simulink model "controller_test"  (R2015a)
settings: Solver=ode5  StartTime=0.0  StopTime=9  FixedStep=1e-4  RelTol=1e-3
values from neighbouring files (symbols this model uses):
  A = A(1:4,1:4)    [main_matlab_version_3.m]    (also in main_matlab_version_4.m)
  B = B(1:4,:)    [main_matlab_version_3.m]    (also in main_matlab_version_4.m)
  C = [-23.1554338545303,9.56281796834669,0.435674513053965,-0.466194198179862]    [finding_Y.m]    (also in main_matlab_version_3.m = C(:,1:4); main_matlab_version_4.m = C(:,1:4))
  E = [0.258916103898922;0.101956592759767;-1.80129126804772;-4.56185147008189]    [finding_Y.m]    (also in main_matlab_version_3.m = E(1:4,:); main_matlab_version_4.m = E(1:4,:))
  H = -E*CEp+Y*(eye(ny,ny)-(C*E)*CEp)    [main_matlab_version_1.m]    (also in main_matlab_version_2.m; main_matlab_version_3.m = H1+Y*H2; main_matlab_version_4.m = H1+Y*H2)
  J = (eye(n,n)+(-E*CEp+Y*(eye(ny,ny)-(C*E)*CEp))*C)*B    [main_matlab_version_1.m]    (also in main_matlab_version_2.m; main_matlab_version_3.m; main_matlab_version_4.m)
  L = K-N*H    [main_matlab_version_2.m]    (also in main_matlab_version_3.m; main_matlab_version_4.m = Q2\Lh)
  N = P*A-K*C    [main_matlab_version_1.m]    (also in main_matlab_version_2.m; main_matlab_version_3.m; main_matlab_version_4.m)
  T = Th/X    [main_matlab_version_1.m]    (also in main_matlab_version_2.m; main_matlab_version_3.m; main_matlab_version_4.m)
libraries: simulink x2
settings Model: Creator=p4wp4w  LastModifiedBy=p4wp4w

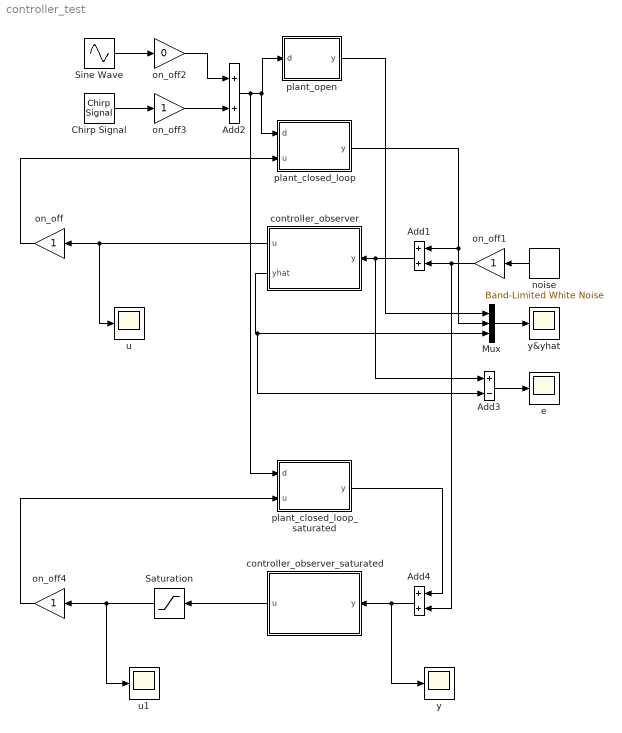
== system controller_test ==
  Add1 : Sum
  Add2 : Sum
  Add3 : Sum  Inputs=+-
  Add4 : Sum
  Chirp Signal : simulink/Sources/Chirp Signal  f1=0.1  T=9  f2=90
  Mux : Mux  Inputs=3
  Saturation : Saturate  UpperLimit=1.5  LowerLimit=-1.5
  Sine Wave : Sin  Frequency=14*2*pi  SampleTime=0
  controller_observer : Subsystem
  controller_observer_saturated : Subsystem
  e : Scope
      settings: ShowLegends=on  YMin=-1.5e+08  YMax=1.75e+08  SaveName=ScopeData2
  noise : simulink/Sources/Band-Limited White Noise  Cov=[1e-12]  Ts=1e-4  seed=[23341]
  on_off{,1,3..4} (4 alike) : Gain
  on_off2 : Gain  Gain=0
  plant_closed_loop : Subsystem
  plant_closed_loop_saturated : Subsystem
  plant_open : Subsystem
  u : Scope
  u1 : Scope
      settings: SaveName=ScopeData3
  y : Scope
      settings: SaveName=ScopeData4
  y&yhat : Scope
      settings: ShowLegends=on  YMin=-1.5e+08  YMax=1.75e+08
  wires:
  noise/1 -> on_off1/1
  Add1/1 -> Add3/1, controller_observer/1(y)
  Mux/1 -> y&yhat/1
  controller_observer/2(yhat) -> Add3/2, Mux/3
  on_off1/1 -> Add1/2, Add4/2
  plant_closed_loop/1(y) -> Mux/2, Add1/1
  on_off/1 -> plant_closed_loop/2(u)
  plant_open/1(y) -> Mux/1
  Sine Wave/1 -> on_off2/1
  Chirp Signal/1 -> on_off3/1
  on_off3/1 -> Add2/2
  on_off2/1 -> Add2/1
  Add2/1 -> plant_closed_loop_saturated/1(d), plant_closed_loop/1(d), plant_open/1(d)
  Add3/1 -> e/1
  controller_observer/1(u) -> u/1, on_off/1
  controller_observer_saturated/1(u) -> Saturation/1
  Saturation/1 -> u1/1, on_off4/1
  Add4/1 -> y/1, controller_observer_saturated/1(y)
  plant_closed_loop_saturated/1(y) -> Add4/1
  on_off4/1 -> plant_closed_loop_saturated/2(u)

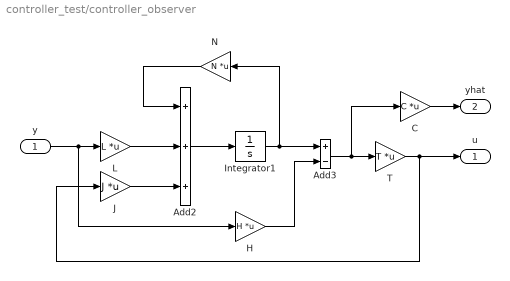
== system controller_test/controller_observer ==
  y : Inport
  Add2 : Sum  Inputs=+++
  Add3 : Sum  Inputs=+-
  C : Gain  Gain=C  Multiplication=Matrix(K*u)
  H : Gain  Gain=H  Multiplication=Matrix(K*u)
  Integrator1 : Integrator
  J : Gain  Gain=J  Multiplication=Matrix(K*u)
  L : Gain  Gain=L  Multiplication=Matrix(K*u)
  N : Gain  Gain=N  Multiplication=Matrix(K*u)
  T : Gain  Gain=T  Multiplication=Matrix(K*u)
  u : Outport
  yhat : Outport  Port=2
  wires:
  H/1 -> Add3/2
  Add3/1 -> C/1, T/1
  L/1 -> Add2/2
  T/1 -> u/1, J/1
  J/1 -> Add2/3
  N/1 -> Add2/1
  Add2/1 -> Integrator1/1
  Integrator1/1 -> Add3/1, N/1
  y/1 -> H/1, L/1
  C/1 -> yhat/1

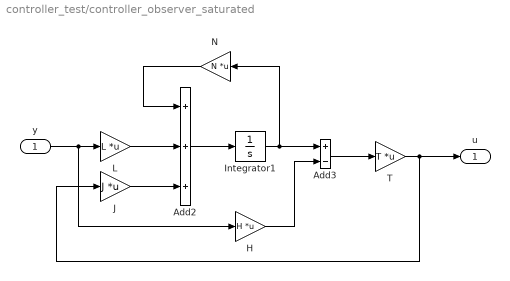
== system controller_test/controller_observer_saturated ==
  y : Inport
  Add2 : Sum  Inputs=+++
  Add3 : Sum  Inputs=+-
  H : Gain  Gain=H  Multiplication=Matrix(K*u)
  Integrator1 : Integrator
  J : Gain  Gain=J  Multiplication=Matrix(K*u)
  L : Gain  Gain=L  Multiplication=Matrix(K*u)
  N : Gain  Gain=N  Multiplication=Matrix(K*u)
  T : Gain  Gain=T  Multiplication=Matrix(K*u)
  u : Outport
  wires:
  y/1 -> L/1, H/1
  Integrator1/1 -> N/1, Add3/1
  Add2/1 -> Integrator1/1
  N/1 -> Add2/1
  J/1 -> Add2/3
  T/1 -> J/1, u/1
  L/1 -> Add2/2
  Add3/1 -> T/1
  H/1 -> Add3/2

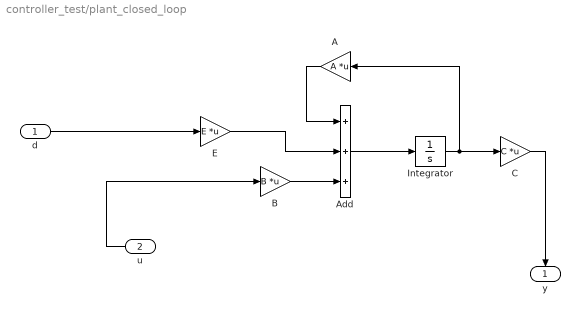
== system controller_test/plant_closed_loop ==
  d : Inport
  u : Inport  Port=2
  A : Gain  Gain=A  Multiplication=Matrix(K*u)
  Add : Sum  Inputs=+++
  B : Gain  Gain=B  Multiplication=Matrix(K*u)
  C : Gain  Gain=C  Multiplication=Matrix(K*u)
  E : Gain  Gain=E  Multiplication=Matrix(K*u)
  Integrator : Integrator
  y : Outport
  wires:
  u/1 -> B/1
  Add/1 -> Integrator/1
  C/1 -> y/1
  E/1 -> Add/2
  A/1 -> Add/1
  B/1 -> Add/3
  d/1 -> E/1
  Integrator/1 -> C/1, A/1

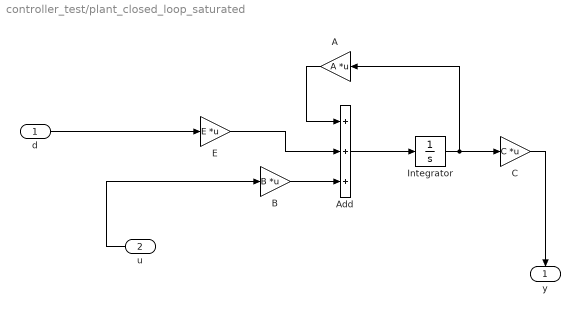
== system controller_test/plant_closed_loop_saturated ==
  d : Inport
  u : Inport  Port=2
  A : Gain  Gain=A  Multiplication=Matrix(K*u)
  Add : Sum  Inputs=+++
  B : Gain  Gain=B  Multiplication=Matrix(K*u)
  C : Gain  Gain=C  Multiplication=Matrix(K*u)
  E : Gain  Gain=E  Multiplication=Matrix(K*u)
  Integrator : Integrator
  y : Outport
  wires:
  Integrator/1 -> A/1, C/1
  d/1 -> E/1
  B/1 -> Add/3
  A/1 -> Add/1
  E/1 -> Add/2
  C/1 -> y/1
  Add/1 -> Integrator/1
  u/1 -> B/1

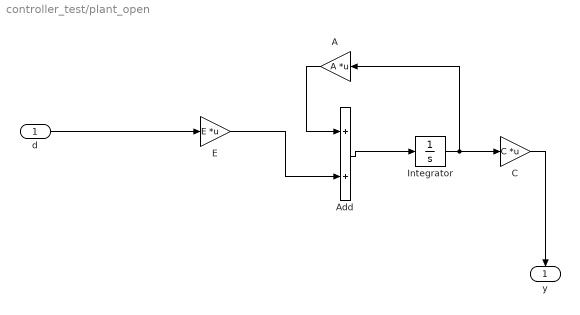
== system controller_test/plant_open ==
  d : Inport
  A : Gain  Gain=A  Multiplication=Matrix(K*u)
  Add : Sum
  C : Gain  Gain=C  Multiplication=Matrix(K*u)
  E : Gain  Gain=E  Multiplication=Matrix(K*u)
  Integrator : Integrator
  y : Outport
  wires:
  Integrator/1 -> A/1, C/1
  d/1 -> E/1
  A/1 -> Add/1
  E/1 -> Add/2
  C/1 -> y/1
  Add/1 -> Integrator/1
